simulink model "BatteryExampleUKF"  (R2017b)
settings: Solver=VariableStepAuto  StartTime=0.0  StopTime=100000  RelTol=1e-3
values from neighbouring files (symbols this model uses):
  C1_LUT = [1913.6 4625.7 23306 10736 18036 12251 9022.9 12447 18872 40764 18721 33630 ... (21 elements, 7x3)]    [BatteryParameters.mat]    (also in RW9_BatteryParameters.mat = [10000 10000 10000 10000 10000 10000 10000 9385.18668996 101)
  Capacity_LUT = [28.0081 27.625 27.6392]    [BatteryParameters.mat]    (also in RW9_BatteryParameters.mat = [2.6 2.55 2.5])
  cell_Cp_heat = 810.5328    [BatteryParameters.mat]    (also in RW9_BatteryParameters.mat = 35.3674127278)
  cell_mass = 1    [BatteryParameters.mat]    (also in RW9_BatteryParameters.mat = 0.0465)
  Em_LUT = [3.4966 3.5519 3.6183 3.7066 3.9131 4.0748 4.1923 3.5057 3.566 3.6337 3.7127 3.9259 ... (21 elements, 7x3)]    [BatteryParameters.mat]    (also in RW9_BatteryParameters.mat = [4 4 4 4 4 4 4 3.59172393305 3.73237152634 3.77937764301 3.8)
  InitCapacity = 30    [BatteryParameters.mat]    (also in RW9_BatteryParameters.mat = 2.6)
  LowerSOC = 0.3    [BatteryParameters.mat]    (also in RW9_BatteryParameters.mat)
  Qe_init = 15.6845    [BatteryParameters.mat]    (also in RW9_BatteryParameters.mat)
  R0_LUT = [0.0117 0.011 0.0114 0.0107 0.0107 0.0113 0.0116 0.0085 0.0085 0.0087 0.0082 0.0083 ... (21 elements, 7x3)]    [BatteryParameters.mat]    (also in RW9_BatteryParameters.mat = [0.1 0.1 0.1 0.1 0.1 0.1 0.1 0.129745781607 0.102359241178 0)
  R1_LUT = [0.0109 0.0069 0.0047 0.0034 0.0033 0.0033 0.0028 0.0029 0.0024 0.0026 0.0016 0.0023 ... (21 elements, 7x3)]    [BatteryParameters.mat]    (also in RW9_BatteryParameters.mat = [0.07 0.07 0.07 0.07 0.07 0.07 0.07 0.0768617046799 0.065453)
  SOC_LUT = [0 0.1 0.25 0.5 0.75 0.9 1]    [BatteryParameters.mat]    (also in RW9_BatteryParameters.mat)
  T_init = 293.15    [BatteryParameters.mat]    (also in RW9_BatteryParameters.mat)
  Temperature_LUT = [278.15 293.15 313.15]    [BatteryParameters.mat]    (also in RW9_BatteryParameters.mat)
  Ts = 1    [BatteryParameters.mat]    (also in RW9_BatteryParameters.mat)
  UpperSOC = 0.9    [BatteryParameters.mat]    (also in RW9_BatteryParameters.mat)
undefined symbols (not defined in the file or in its folder): DiscIntNeverNeededParam, Discrete, sigbuilder_block, Time
libraries: fl_lib x13, nesl_utility x8, simulink x5, ctrlSharedLib x1, sharedTrackingLibrary x1
settings Model: Creator=The MathWorks, Inc.  LastModifiedBy=imrenagi
settings CodeAppCC: StateflowObjectComments=on
settings SimscapeCC: SimscapeNormalizeSystem=off

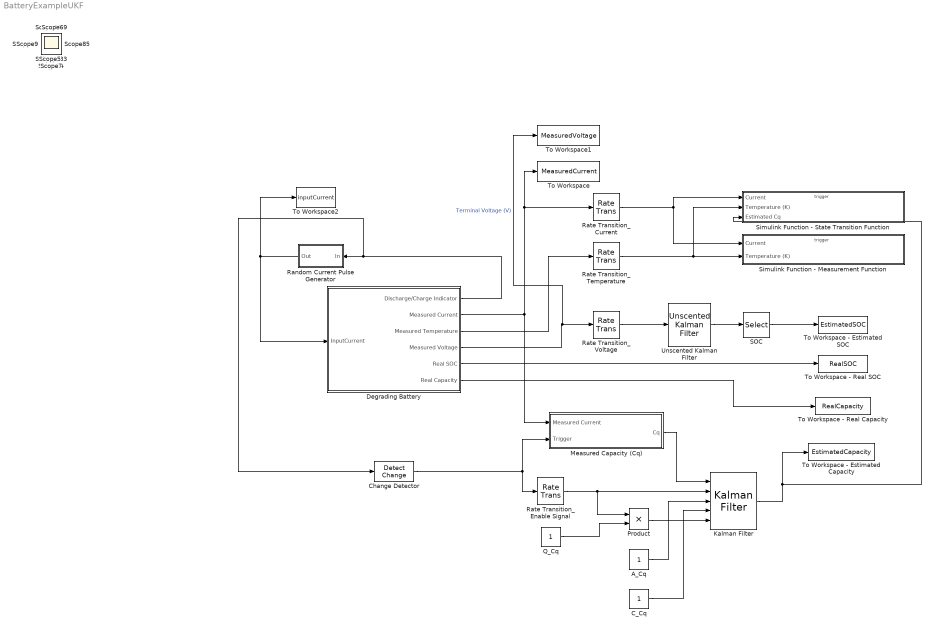
== system BatteryExampleUKF ==
  A_Cq : Constant
  C_Cq : Constant
  Change Detector : simulink/Logic and Bit Operations/Detect Change  vinit=-1  OutDataTypeStr=boolean
  Degrading Battery : Subsystem
  Kalman Filter : ctrlSharedLib/Kalman Filter  TimeDomain=Discrete-Time  UseCurrentEstimator=on  ModelSource=Input port  ModelSourceVariable=ss(0.95,1,1,0,1)  A=1  B=1  C=1  D=0  NumberOfStates=1  NumberOfInputs=1  NumberOfOutputs=1  InitialEstimateSource=Dialog  X0=2.6  P0=0.05  UseK=off  UseGH=off  NumberOfProcessNoiseInputs=1  G=1  TimeInvariantG=on  H=0  TimeInvariantH=on  Q=1  TimeInvariantQ=off  R=0.001  TimeInvariantR=on  N=0  TimeInvariantN=on  AddInputPort=off  AddEnablePort=on  OutputEstimatedY=off  OutputP=off  Ts=Ts
      settings: SourceProductBaseCode=CT
  Measured Capacity (Cq) : Subsystem
  Product : Product
  Q_Cq : Constant
  Random Current Pulse Generator : Subsystem
  Rate Transition_Current : RateTransition  OutPortSampleTime=Ts
  Rate Transition_Enable Signal : RateTransition  OutPortSampleTime=Ts
  Rate Transition_Temperature : RateTransition  InitialCondition=300  OutPortSampleTime=Ts
  Rate Transition_Voltage : RateTransition  InitialCondition=4  OutPortSampleTime=Ts
  SOC : Selector  InputPortWidth=2  IndexOptions=Index vector (dialog)  Indices=1  OutputSizes=1
  Simulink Function - Measurement Function : Subsystem  TreatAsAtomicUnit=on
  Simulink Function - State Transition Function : Subsystem  TreatAsAtomicUnit=on
  To Workspace : ToWorkspace  VariableName=MeasuredCurrent  SaveFormat=Timeseries  SampleTime=-1
  To Workspace - Estimated Capacity : ToWorkspace  VariableName=EstimatedCapacity  SaveFormat=Timeseries  SampleTime=-1
  To Workspace - Estimated SOC : ToWorkspace  VariableName=EstimatedSOC  SaveFormat=Timeseries  SampleTime=-1
  To Workspace - Real Capacity : ToWorkspace  VariableName=RealCapacity  SaveFormat=Timeseries  SampleTime=-1
  To Workspace - Real SOC : ToWorkspace  VariableName=RealSOC  SaveFormat=Timeseries  SampleTime=-1
  To Workspace1 : ToWorkspace  VariableName=MeasuredVoltage  SaveFormat=Timeseries  SampleTime=-1
  To Workspace2 : ToWorkspace  VariableName=inputCurrent  SaveFormat=Timeseries  SampleTime=-1
  Unscented Kalman Filter : sharedTrackingLibrary/Unscented Kalman Filter  StateTransitionFcn=batteryStateFcn  HasAdditiveProcessNoise=Additive  ProcessNoise=diag([2e-8, 3e-7])  HasTimeVaryingProcessNoise=off  HasStateTransitionFcnExtraArgument=0  InitialState=[1; 0]  InitialStateCovariance=diag([0.01, 1])  Alpha=1  Beta=2  Kappa=0  MeasurementFcn1=batteryMeasurementFcn  HasMeasurementEnablePort1=off  HasAdditiveMeasurementNoise1=Additive  MeasurementNoise1=1e-3  HasTimeVaryingMeasurementNoise1=off  HasMeasurementFcnExtraArgument1=0  MeasurementFcn2=myMeasurementFcn  HasMeasurementEnablePort2=off  HasAdditiveMeasurementNoise2=Additive  MeasurementNoise2=1  HasTimeVaryingMeasurementNoise2=off  HasMeasurementFcnExtraArgument2=0  MeasurementFcn3=myMeasurementFcn  HasMeasurementEnablePort3=off  HasAdditiveMeasurementNoise3=Additive  MeasurementNoise3=1  HasTimeVaryingMeasurementNoise3=off  HasMeasurementFcnExtraArgument3=0  MeasurementFcn4=myMeasurementFcn  HasMeasurementEnablePort4=off  HasAdditiveMeasurementNoise4=Additive  MeasurementNoise4=1  HasTimeVaryingMeasurementNoise4=off  HasMeasurementFcnExtraArgument4=0  MeasurementFcn5=myMeasurementFcn  HasMeasurementEnablePort5=off  HasAdditiveMeasurementNoise5=Additive  MeasurementNoise5=1  HasTimeVaryingMeasurementNoise5=off  HasMeasurementFcnExtraArgument5=0  EnableMultirate=off  StateTransitionFcnSampleTime=-1  MeasurementFcn1SampleTime=-1  MeasurementFcn2SampleTime=-1  MeasurementFcn3SampleTime=-1  MeasurementFcn4SampleTime=-1  MeasurementFcn5SampleTime=-1  UseCurrentEstimator=on  OutputStateCovariance=off  DataType=double  SampleTime=Ts  NumberOfMeasurements=1
      settings: SourceProductName=Control System Toolbox  SourceProductBaseCode=CT
  Scope{,1..11,13,17..18,20,22..35} (30 alike) : Scope
  wires:
  Degrading Battery/2(Measured Current) -> Measured Capacity (Cq)/1(Measured Current), To Workspace/1, Rate Transition_Current/1
  Rate Transition_Current/1 -> Simulink Function - Measurement Function/1(Current), Simulink Function - State Transition Function/1(Current)
  Unscented Kalman Filter/1 -> SOC/1
  Rate Transition_Voltage/1 -> Unscented Kalman Filter/1
  Rate Transition_Temperature/1 -> Simulink Function - State Transition Function/2(Temperature (K)), Simulink Function - Measurement Function/2(Temperature (K))
  Degrading Battery/1(Discharge/Charge Indicator) -> Change Detector/1, Random Current Pulse Generator/1(In)
  Random Current Pulse Generator/1(Out) -> To Workspace2/1, Degrading Battery/1(InputCurrent)
  SOC/1 -> To Workspace - Estimated SOC/1
  Degrading Battery/5(Real SOC) -> To Workspace - Real SOC/1
  Measured Capacity (Cq)/1(Cq) -> Kalman Filter/1
  Change Detector/1 -> Measured Capacity (Cq)/2(Trigger), Rate Transition_Enable Signal/1
  Kalman Filter/1 -> To Workspace - Estimated Capacity/1, Simulink Function - State Transition Function/3(Estimated Cq)
  Rate Transition_Enable Signal/1 -> Product/1, Kalman Filter/2
  Degrading Battery/3(Measured Temperature) -> Rate Transition_Temperature/1
  Degrading Battery/4(Measured Voltage) -> To Workspace1/1, Rate Transition_Voltage/1  "Terminal Voltage (V)"
  Product/1 -> Kalman Filter/5
  Q_Cq/1 -> Product/2
  A_Cq/1 -> Kalman Filter/3
  C_Cq/1 -> Kalman Filter/4
  Degrading Battery/6(Real Capacity) -> To Workspace - Real Capacity/1

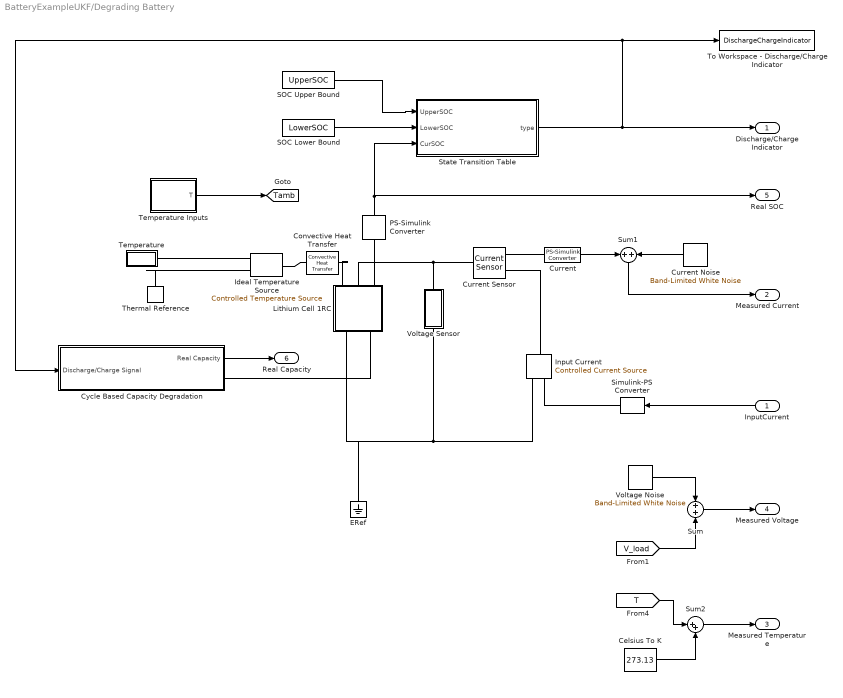
== system BatteryExampleUKF/Degrading Battery ==
  InputCurrent : Inport
  Celsius To K : Constant  Value=273.13
  Convective Heat Transfer : fl_lib/Thermal/Thermal Elements/Convective Heat Transfer  area=cell_area m^2  heat_tr_coeff=h_conv W/(m^2 * K)  T_specify=off  T_priority=High  T=0 K  T_nominal_specify=off  T_nominal_unit=K  T_nominal_value=1  Q_specify=off  Q_priority=High  Q=0 J/s  Q_nominal_specify=off  Q_nominal_unit=J/s  Q_nominal_value=1
  Current : nesl_utility/PS-Simulink Converter  PhysicalDomain=network_engine_domain  SubClassName=ps_output  LeftPortType=input  RightPortType=output  PseudoPeriodic=off  Frequencies=[]  Unit=1  AffineConversion=off
  Current Noise : simulink/Sources/Band-Limited White Noise  Cov=2.5e-2  Ts=Ts  seed=[1234]
  Current Sensor : fl_lib/Electrical/Electrical Sensors/Current Sensor
  Cycle Based Capacity Degradation : Subsystem
  ERef : fl_lib/Electrical/Electrical Elements/Electrical Reference
  Ideal Temperature Source : fl_lib/Thermal/Thermal Sources/Controlled Temperature Source
      settings: SourceProductName=Simscape
  Input Current : fl_lib/Electrical/Electrical Sources/Controlled Current Source
  Lithium Cell 1RC : Subsystem  Tag=PublishSubsystemCustomStyle  mask(Lithium cell (one RC-branch equivalent circuit)){Qe_init=Qe_init, T_init=T_init, Capacity_LUT=Capacity_LUT, Em_LUT=Em_LUT, R0_LUT=R0_LUT, R1_LUT=R1_LUT, C1_LUT=C1_LUT, cell_mass=cell_mass, cell_Cp_heat=cell_Cp_heat, SOC_LUT=SOC_LUT, Temperature_LUT=Temperature_LUT}
      mask prompts: Qe_init "Initial charge deficit (A*hr)"; T_init "Initial cell temperature (K)"; Capacity_LUT "Capacity (A*hr, 1xN table)"; Em_LUT "Em open-circuit voltage (volts, MxN table)"; R0_LUT "R0 terminal resistance (ohms, MxN table)"; R1_LUT "R1 resistance (ohms, MxN table)"; C1_LUT "C1 capacitance (farads, MxN table)"; cell_mass "Cell mass (kg)"; cell_Cp_heat "Cell specific heat (J/kg/K)"; SOC_LUT "SOC table breakpoints (Mx1 array)"; Temperature_LUT "Temperature table breakpoints (K, 1xN array)"
      mask DialogControl ParameterTabVar0 Prompt: Initial Conditions
      mask DialogControl ParameterTabVar01 Prompt: Electrical
      mask DialogControl ParameterTabVar012 Prompt: Thermal
      mask DialogControl ParameterTabVar0123 Prompt: Table Breakpoints
      mask Display:
      | % Battery icon
      | plot([0 0],[-1.5 -0.4])
      | plot([0 0 0.8 0.8],[0.2 0.9 0.9 1.5])
      | patch([-1 1 1 -1]*0.4,[1 1 -1 -1]*0.15-0.5,[0;0;0]);
      | patch([-1 1 1 -1]*0.9,[1 1 -1 -1]*0.15+0.1,[0;0;0]);
      | 
      | % Thermal port
      | plot([-1.2,-1.2],[0.5,0.9])
      | plot([-0.4,-0.4],[0.5,0.9])
      | plot([-0.8,-0.8],[0.9,1.5])
      | plot(0.35*cos(0:2*pi/50:2*pi)-0.8,0.15*sin(0:2*pi/50:2*pi)+0.85)
      | plot(0.35*cos(pi:2*pi/50:2*pi)-0.8,0.15*sin(pi:2*pi/50:2*pi)+0.55)
      | 
      | % Plot points to set plot range
      | color('white');plot(1.5,1.5);plot(-1.5,-1.5)
      | 
      | color('red')
      | port_label('LConn',1,'H')
      | port_label('LConn',2,'+')
      | port_label('RConn',1,'-')
  PS-Simulink Converter : nesl_utility/PS-Simulink Converter  PhysicalDomain=network_engine_domain  SubClassName=ps_output  LeftPortType=input  RightPortType=output  PseudoPeriodic=off  Frequencies=[]  Unit=1  AffineConversion=off
  SOC Lower Bound : Constant  Value=LowerSOC
  SOC Upper Bound : Constant  Value=UpperSOC
  Simulink-PS Converter : nesl_utility/Simulink-PS Converter  PhysicalDomain=network_engine_domain  SubClassName=ps_input  LeftPortType=input  RightPortType=output  PseudoPeriodic=off  Frequencies=[]  NoiseDistribution=none  NoiseParameters=[]  Unit=A  AffineConversion=off  FilteringAndDerivatives=zero  SimscapeFilterOrder=1  InputFilterTimeConstant=.001  UdotUserProvided=1
  State Transition Table : State Transition Table  TreatAsAtomicUnit=on
  Sum : Sum
  Sum1 : Sum
  Sum2 : Sum  Inputs=|++
  Temperature : Subsystem
      mask Display: disp('Tamb')
  Temperature Inputs : Subsystem
  Thermal Reference : fl_lib/Thermal/Thermal Elements/Thermal Reference
  To Workspace - Discharge/Charge Indicator : ToWorkspace  VariableName=DischargeChargeIndicator  SaveFormat=Timeseries  SampleTime=-1
  Voltage Sensor : Subsystem
      mask Display: disp('V_load')
  Voltage Noise : simulink/Sources/Band-Limited White Noise  Cov=1.5e-3  Ts=Ts  seed=[1234]
  Discharge/Charge Indicator : Outport
  Measured Current : Outport  Port=2
  Measured Temperature : Outport  Port=3
  Measured Voltage : Outport  Port=4
  Real SOC : Outport  Port=5
  Real Capacity : Outport  Port=6
  tag scope: Tamb=global
  wires:
  SOC Lower Bound/1 -> State Transition Table/2(LowerSOC)
  SOC Upper Bound/1 -> State Transition Table/1(UpperSOC)
  PS-Simulink Converter/1 -> State Transition Table/3(CurSOC), Real SOC/1
  Temperature Inputs/1(T) -> [Tamb]
  State Transition Table/1(type) -> To Workspace - Discharge/Charge Indicator/1, Cycle Based Capacity Degradation/1(Discharge/Charge Signal), Discharge/Charge Indicator/1
  [V_load] -> Sum/2
  Sum/1 -> Measured Voltage/1
  InputCurrent/1 -> Simulink-PS Converter/1
  Sum1/1 -> Measured Current/1
  Current/1 -> Sum1/1
  Current Noise/1 -> Sum1/2
  Celsius To K/1 -> Sum2/2
  Sum2/1 -> Measured Temperature/1
  [T] -> Sum2/1
  Cycle Based Capacity Degradation/1(Real Capacity) -> Real Capacity/1
  Voltage Noise/1 -> Sum/1
  connections:
  Lithium Cell 1RC/LConn1 -- Convective Heat Transfer/RConn1
  Current Sensor/RConn2 -- Input Current/LConn1
  Voltage Sensor/RConn1 -- Input Current/RConn2 -- ERef/LConn1 -- Lithium Cell 1RC/RConn1
  Lithium Cell 1RC/LConn3 -- PS-Simulink Converter/LConn1
  Current Sensor/LConn1 -- Lithium Cell 1RC/LConn2 -- Voltage Sensor/LConn1
  Current/LConn1 -- Current Sensor/RConn1
  Ideal Temperature Source/RConn1 -- Temperature/LConn1
  Ideal Temperature Source/RConn2 -- Thermal Reference/LConn1
  Simulink-PS Converter/RConn1 -- Input Current/RConn1
  Cycle Based Capacity Degradation/RConn1 -- Lithium Cell 1RC/RConn2
  Ideal Temperature Source/LConn1 -- Convective Heat Transfer/LConn1

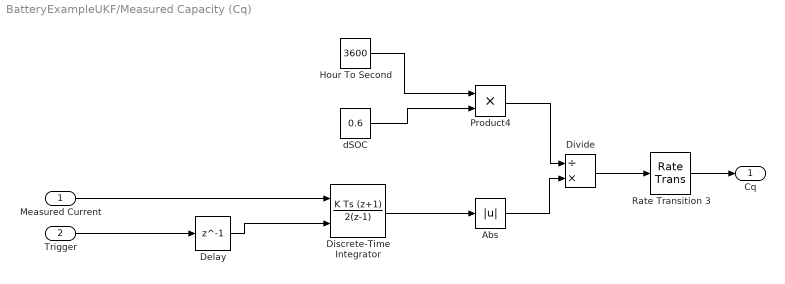
== system BatteryExampleUKF/Measured Capacity (Cq) ==
  Measured Current : Inport
  Trigger : Inport  Port=2
  Abs : Abs
  Delay : Delay  DelayLength=1  InitialCondition=0
  Discrete-Time Integrator : DiscreteIntegrator  IntegratorMethod=Integration: Trapezoidal  ExternalReset=rising  InitialConditionSetting=State (most efficient)  SampleTime=-1  ICPrevOutput=DiscIntNeverNeededParam  ICPrevScaledInput=DiscIntNeverNeededParam
  Divide : Product  Inputs=/*
  Hour To Second : Constant  Value=3600
  Product4 : Product
  Rate Transition 3 : RateTransition  InitialCondition=InitCapacity  OutPortSampleTime=Ts
  dSOC : Constant  Value=0.6
  Cq : Outport
  wires:
  Measured Current/1 -> Discrete-Time Integrator/1
  Abs/1 -> Divide/2
  Discrete-Time Integrator/1 -> Abs/1
  Product4/1 -> Divide/1
  Delay/1 -> Discrete-Time Integrator/2
  Hour To Second/1 -> Product4/1
  Trigger/1 -> Delay/1
  dSOC/1 -> Product4/2
  Rate Transition 3/1 -> Cq/1
  Divide/1 -> Rate Transition 3/1

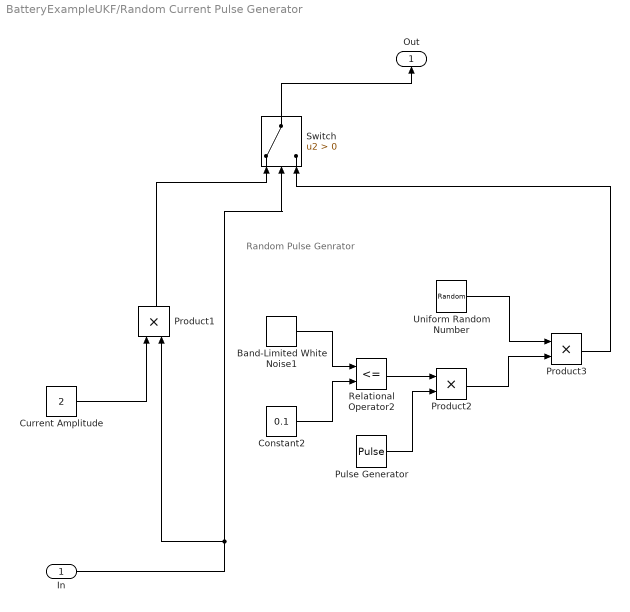
== system BatteryExampleUKF/Random Current Pulse Generator ==
  note: Random Pulse Genrator
  In : Inport
  Band-Limited White Noise1 : simulink/Sources/Band-Limited White Noise  Cov=0.1  Ts=50  seed=[23341]
  Constant2 : Constant  Value=0.1
  Current Amplitude : Constant  Value=2
  Product1 : Product
  Product2 : Product
  Product3 : Product
  Pulse Generator : DiscretePulseGenerator  PulseType=Time based  Amplitude=-1  Period=1000  PulseWidth=90
  Relational Operator2 : RelationalOperator  Operator=<=  OutDataTypeStr=boolean  RndMeth=Simplest
  Switch : Switch  Criteria=u2 > Threshold
  Uniform Random Number : UniformRandomNumber  Minimum=0.7  Maximum=1.5  SampleTime=100
  Out : Outport
  wires:
  In/1 -> Product1/2, Switch/2
  Constant2/1 -> Relational Operator2/2
  Band-Limited White Noise1/1 -> Relational Operator2/1
  Pulse Generator/1 -> Product2/2
  Relational Operator2/1 -> Product2/1
  Uniform Random Number/1 -> Product3/1
  Product2/1 -> Product3/2
  Product1/1 -> Switch/1
  Current Amplitude/1 -> Product1/1
  Product3/1 -> Switch/3
  Switch/1 -> Out/1

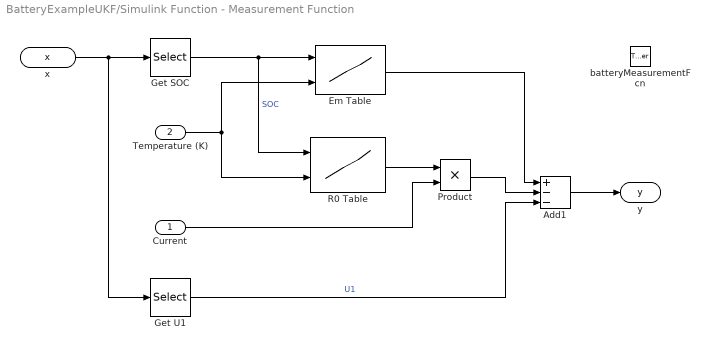
== system BatteryExampleUKF/Simulink Function - Measurement Function ==
  Current : Inport
  Temperature (K) : Inport  Port=2
  batteryMeasurementFcn : TriggerPort  TriggerType=function-call  IsSimulinkFunction=on  FunctionName=batteryMeasurementFcn  VariantControl=Variant
  Add1 : Sum  Inputs=+--
  Em Table : Lookup_n-D  BreakpointsForDimension1=SOC_LUT  BreakpointsForDimension2=Temperature_LUT  Table=Em_LUT  InternalRulePriority=Speed  RndMeth=Simplest  InputSameDT=on
  Get SOC : Selector  InputPortWidth=2  IndexOptions=Index vector (dialog)  Indices=[1]  OutputSizes=1
  Get U1 : Selector  InputPortWidth=2  IndexOptions=Index vector (dialog)  Indices=2  OutputSizes=1
  Product : Product
  R0 Table : Lookup_n-D  BreakpointsForDimension1=SOC_LUT  BreakpointsForDimension2=Temperature_LUT  Table=R0_LUT  InternalRulePriority=Speed  RndMeth=Simplest  InputSameDT=on
  x : ArgIn  DisableCoverage=on  PortDimensions=2  ArgumentName=x
  y : ArgOut  DisableCoverage=on  ArgumentName=y
  wires:
  x/1 -> Get U1/1, Get SOC/1
  Get SOC/1 -> R0 Table/1, Em Table/1  "SOC"
  Em Table/1 -> Add1/1
  Add1/1 -> y/1
  Temperature (K)/1 -> R0 Table/2, Em Table/2
  R0 Table/1 -> Product/1
  Current/1 -> Product/2
  Product/1 -> Add1/2
  Get U1/1 -> Add1/3  "U1"

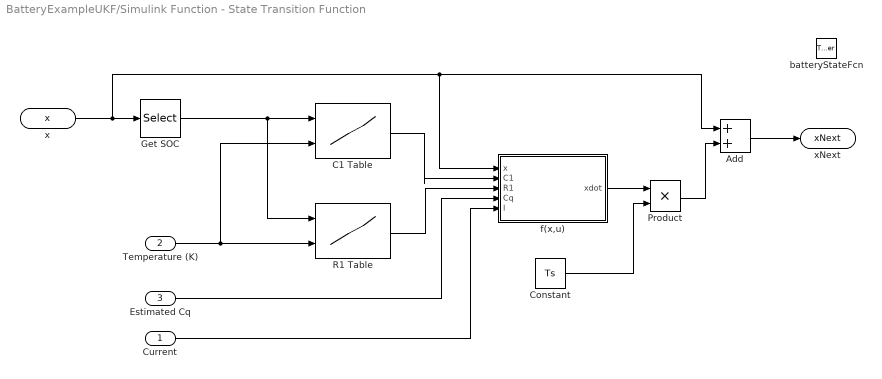
== system BatteryExampleUKF/Simulink Function - State Transition Function ==
  Current : Inport
  Temperature (K) : Inport  Port=2
  Estimated Cq : Inport  Port=3
  batteryStateFcn : TriggerPort  TriggerType=function-call  IsSimulinkFunction=on  FunctionName=batteryStateFcn  VariantControl=Variant
  Add : Sum
  C1 Table : Lookup_n-D  BreakpointsForDimension1=SOC_LUT  BreakpointsForDimension2=Temperature_LUT  Table=C1_LUT  InternalRulePriority=Speed  RndMeth=Simplest  InputSameDT=on
  Constant : Constant  Value=Ts
  Get SOC : Selector  InputPortWidth=2  IndexOptions=Index vector (dialog)  Indices=1  OutputSizes=1
  Product : Product
  R1 Table : Lookup_n-D  BreakpointsForDimension1=SOC_LUT  BreakpointsForDimension2=Temperature_LUT  Table=R1_LUT  InternalRulePriority=Speed  RndMeth=Simplest  InputSameDT=on
  f(x,u) : MATLAB Function  TreatAsAtomicUnit=on
  x : ArgIn  DisableCoverage=on  PortDimensions=2  ArgumentName=x
  xNext : ArgOut  DisableCoverage=on  PortDimensions=2  ArgumentName=xNext
  wires:
  x/1 -> f(x,u)/1(x), Add/1, Get SOC/1
  Add/1 -> xNext/1
  Temperature (K)/1 -> C1 Table/2, R1 Table/2
  Get SOC/1 -> R1 Table/1, C1 Table/1
  C1 Table/1 -> f(x,u)/2(C1)
  R1 Table/1 -> f(x,u)/3(R1)
  Current/1 -> f(x,u)/5(I)
  Constant/1 -> Product/2
  f(x,u)/1(xdot) -> Product/1
  Product/1 -> Add/2
  Estimated Cq/1 -> f(x,u)/4(Cq)

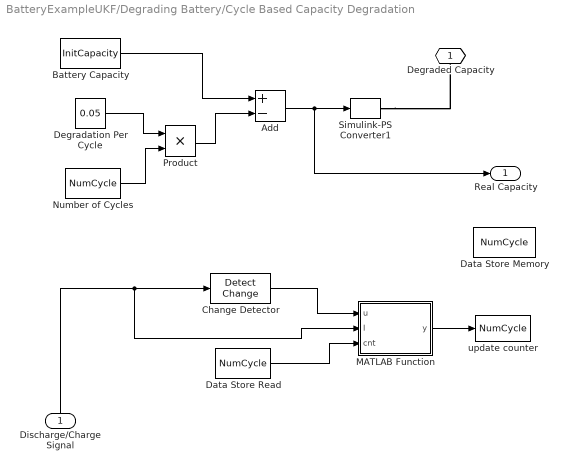
== system BatteryExampleUKF/Degrading Battery/Cycle Based Capacity Degradation ==
  Discharge/Charge Signal : Inport
  Add : Sum  Inputs=+-
  Battery Capacity : Constant  Value=InitCapacity
  Change Detector : simulink/Logic and Bit Operations/Detect Change  vinit=-1  OutDataTypeStr=boolean
  Data Store Memory : DataStoreMemory  DataStoreName=NumCycle  ShowAdditionalParam=off
  Data Store Read : DataStoreRead  DataStoreName=NumCycle
  Degradation Per Cycle : Constant  Value=0.05
  MATLAB Function : MATLAB Function  TreatAsAtomicUnit=on
  Number of Cycles : DataStoreRead  DataStoreName=NumCycle
  Product : Product
  Simulink-PS Converter1 : nesl_utility/Simulink-PS Converter  PhysicalDomain=network_engine_domain  SubClassName=ps_input  LeftPortType=input  RightPortType=output  PseudoPeriodic=off  Frequencies=[]  NoiseDistribution=none  NoiseParameters=[]  Unit=hr*A  AffineConversion=off  FilteringAndDerivatives=zero  SimscapeFilterOrder=1  InputFilterTimeConstant=.001  UdotUserProvided=1
  update counter : DataStoreWrite  DataStoreName=NumCycle
  Degraded Capacity : PMIOPort  Port=1  Side=Right
  Real Capacity : Outport
  wires:
  Add/1 -> Real Capacity/1, Simulink-PS Converter1/1
  Degradation Per Cycle/1 -> Product/1
  MATLAB Function/1(y) -> update counter/1
  Battery Capacity/1 -> Add/1
  Change Detector/1 -> MATLAB Function/1(u)
  Number of Cycles/1 -> Product/2
  Product/1 -> Add/2
  Data Store Read/1 -> MATLAB Function/3(cnt)
  Discharge/Charge Signal/1 -> Change Detector/1, MATLAB Function/2(I)
  connections:
  Simulink-PS Converter1/RConn1 -- Degraded Capacity/RConn1

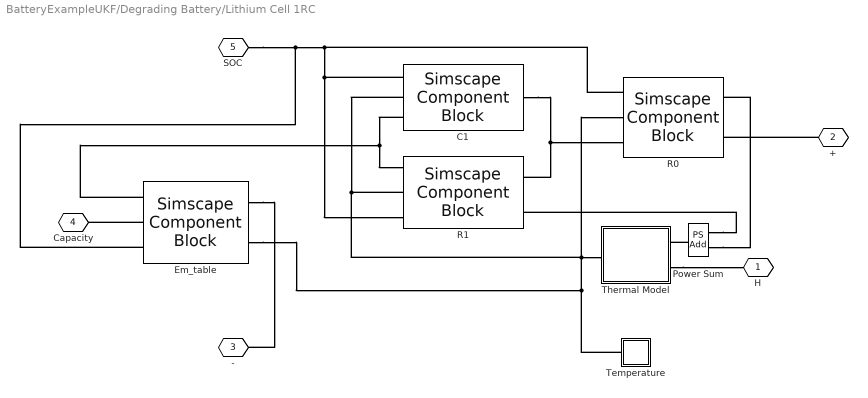
== system BatteryExampleUKF/Degrading Battery/Lithium Cell 1RC ==
  C1 : SimscapeComponentBlock  SourceFile=C_table  ComponentPath=C_table  ComponentVariants=C_table  ComponentVariantNames=C_table  ClassName=C_table  SchemaVersion=1  C_Table=C1_LUT F  SOC_Table=SOC_LUT  Temp_Table=Temperature_LUT K  v0=0 V
      settings: CopyFcn=simscape.engine.sli.internal.componentblockcallback(gcbh,'COPY')  PreCopyFcn=simscape.engine.sli.internal.componentblockcallback(gcbh,'PRECOPY')  PreDeleteFcn=simscape.engine.sli.internal.componentblockcallback(gcbh,'PREDELETE')
      mask Type: C_table
      mask Display:
      | disp('Simscape\n\n\n')
      | disp('\n\n\nC_table');
      | color('red');
      | port_label('LConn', 3,'SOC');
      | port_label('LConn', 2,'T');
      | port_label('RConn', 1,'-');
      | port_label('LConn', 1,'+');
  Em_table : SimscapeComponentBlock  SourceFile=Em_table  ComponentPath=Em_table  ComponentVariants=Em_table  ComponentVariantNames=Em_table  ClassName=Em_table  SchemaVersion=1  Em_Table=Em_LUT V  SOC_Table=SOC_LUT  Temp_Table=Temperature_LUT K  Qinit=Qinit hr*A
      settings: CopyFcn=simscape.engine.sli.internal.componentblockcallback(gcbh,'COPY')  PreCopyFcn=simscape.engine.sli.internal.componentblockcallback(gcbh,'PRECOPY')  PreDeleteFcn=simscape.engine.sli.internal.componentblockcallback(gcbh,'PREDELETE')
      mask Type: Em_table
      mask Display:
      | disp('Simscape\n\n\n')
      | disp('\n\n\nEm_table');
      | color('red');
      | port_label('LConn', 3,'SOC');
      | port_label('LConn', 2,'Capacity');
      | port_label('RConn', 2,'T');
      | port_label('RConn', 1,'-');
      | port_label('LConn', 1,'+');
  Power Sum : fl_lib/Physical Signals/Functions/PS Add
  R0 : SimscapeComponentBlock  SourceFile=R_table  ComponentPath=R_table  ComponentVariants=R_table  ComponentVariantNames=R_table  ClassName=R_table  SchemaVersion=1  R_Table=R0_LUT Ohm  SOC_Table=SOC_LUT  Temp_Table=Temperature_LUT K
      settings: CopyFcn=simscape.engine.sli.internal.componentblockcallback(gcbh,'COPY')  PreCopyFcn=simscape.engine.sli.internal.componentblockcallback(gcbh,'PRECOPY')  PreDeleteFcn=simscape.engine.sli.internal.componentblockcallback(gcbh,'PREDELETE')
      mask Type: R_table
      mask Display:
      | disp('Simscape\n\n\n')
      | disp('\n\n\nR_table');
      | color('red');
      | port_label('RConn', 2,'POW');
      | port_label('LConn', 3,'SOC');
      | port_label('LConn', 2,'T');
      | port_label('RConn', 1,'-');
      | port_label('LConn', 1,'+');
  R1 : SimscapeComponentBlock  SourceFile=R_table  ComponentPath=R_table  ComponentVariants=R_table  ComponentVariantNames=R_table  ClassName=R_table  SchemaVersion=1  R_Table=R1_LUT Ohm  SOC_Table=SOC_LUT  Temp_Table=Temperature_LUT K
      settings: CopyFcn=simscape.engine.sli.internal.componentblockcallback(gcbh,'COPY')  PreCopyFcn=simscape.engine.sli.internal.componentblockcallback(gcbh,'PRECOPY')  PreDeleteFcn=simscape.engine.sli.internal.componentblockcallback(gcbh,'PREDELETE')
      mask Type: R_table
      mask Display:
      | disp('Simscape\n\n\n')
      | disp('\n\n\nR_table');
      | color('red');
      | port_label('RConn', 2,'POW');
      | port_label('LConn', 3,'SOC');
      | port_label('LConn', 2,'T');
      | port_label('RConn', 1,'-');
      | port_label('LConn', 1,'+');
  Temperature : Subsystem
  Thermal Model : Subsystem
  H : PMIOPort  Tag=PMCPort  Port=1  Side=Left
  + : PMIOPort  Tag=PMCPort  Port=2  Side=Left
  - : PMIOPort  Tag=PMCPort  Port=3  Side=Right
  Capacity : PMIOPort  Tag=PMCPort  Port=4  Side=Right
  SOC : PMIOPort  Tag=PMCPort  Port=5  Side=Left
  connections:
  R0/LConn3 -- Em_table/LConn3 -- SOC/RConn1 -- R1/LConn3 -- C1/LConn3
  Thermal Model/LConn2 -- H/RConn1
  Em_table/RConn1 -- -/RConn1
  +/RConn1 -- R0/RConn1
  C1/LConn1 -- R1/LConn1 -- Em_table/LConn1
  Power Sum/LConn2 -- R1/RConn2
  R0/LConn2 -- Em_table/RConn2 -- Temperature/LConn1 -- Thermal Model/RConn1 -- R1/LConn2 -- C1/LConn2
  Power Sum/RConn1 -- Thermal Model/LConn1
  C1/RConn1 -- R1/RConn1 -- R0/LConn1
  Power Sum/LConn1 -- R0/RConn2
  Em_table/LConn2 -- Capacity/RConn1

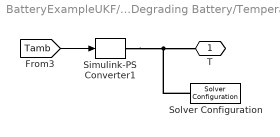
== system BatteryExampleUKF/Degrading Battery/Temperature ==
  Simulink-PS Converter1 : nesl_utility/Simulink-PS Converter  PhysicalDomain=network_engine_domain  SubClassName=ps_input  LeftPortType=input  RightPortType=output  PseudoPeriodic=off  Frequencies=[]  NoiseDistribution=none  NoiseParameters=[]  Unit=degC  AffineConversion=on  FilteringAndDerivatives=zero  SimscapeFilterOrder=1  InputFilterTimeConstant=.001  UdotUserProvided=1
  Solver Configuration : nesl_utility/Solver Configuration  PhysicalDomain=network_engine_domain  SubClassName=solver  LeftPortType=input  RightPortType=generic  Accelerate=off  Tones=[]  Harmonics=[]  SimulateNoise=off  Profile=off  UseLocalSampling=off  EnableSwitchedLinearOptims=on  FrequencyDomain=off  UseCCode=off  RelTol=0.001  AbsTol=1e-06  MinStep=1e-09  ToWorkspace=off  RevertToSquareIcSolve=off  NumHomotopyIterations=100  PhasorMode=off  PhasorModeNumHarmonics=1  DoDC=off  ResidualTolerance=1e-9  UseLocalSolver=off  LocalSolverChoice=NE_BACKWARD_EULER_ADVANCER  LocalSolverSampleTime=1  DoFixedCost=off  MaxNonlinIter=3  MaxModeIter=2  LinearAlgebra=Sparse  DelaysMemoryBudget=1024  AutomaticFiltering=on  FilteringTimeConstant=0.001
  T : PMIOPort  Port=1  Side=Left
  wires:
  [Tamb] -> Simulink-PS Converter1/1
  connections:
  Simulink-PS Converter1/RConn1 -- Solver Configuration/RConn1 -- T/RConn1

== system BatteryExampleUKF/Degrading Battery/Temperature Inputs ==
  Signal Builder : Subsystem  Tag=STV Subsys  LoadFcn=sigbuilder_block('load');  StartFcn=sigbuilder_block('start');  StopFcn=sigbuilder_block('stop');  ClipboardFcn=sigbuilder_block('clipboard');  mask(Sigbuilder block){tuvar=[0:10]}
      mask help: Simulink:masks:SigbuilderBlock_MD
      mask init:
      | if ~strcmp(get_param(bdroot(gcbh),'SimulationStatus'),'stopped') tuvar = sigbuilder_block('maskInit'); end
      settings: CopyFcn=sigbuilder_block('copy');  DeleteFcn=sigbuilder_block('delete');  ModelCloseFcn=sigbuilder_block('modelClose');  PreSaveFcn=sigbuilder_block('preSave');  PauseFcn=sigbuilder_block('pause');  ContinueFcn=sigbuilder_block('continue');  NameChangeFcn=sigbuilder_block('namechange');  OpenFcn=sigbuilder_block('open',[45.75 269.25 978 385.5 ]);  CloseFcn=sigbuilder_block('close');
      mask Display: plot(0, 0, 100, 100,[2, 2, 32, 32, 2], [68, 8, 8, 68, 68],[32, 2], [38, 38], [32, 19, 2],[53, 60, 44], [32, 17, 17, 2],[16, 16, 31, 31]);txt = getActiveGroup(gcbh);text(2, 100, txt,'verticalAlignment', 'top');
  T : Outport
  wires:
  Signal Builder/1(Ambient Temp) -> T/1

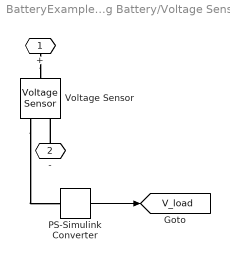
== system BatteryExampleUKF/Degrading Battery/Voltage Sensor ==
  PS-Simulink Converter : nesl_utility/PS-Simulink Converter  PhysicalDomain=network_engine_domain  SubClassName=ps_output  LeftPortType=input  RightPortType=output  PseudoPeriodic=off  Frequencies=[]  Unit=V  AffineConversion=off
  Voltage Sensor : fl_lib/Electrical/Electrical Sensors/Voltage Sensor
  + : PMIOPort  Port=1  Side=Left
  - : PMIOPort  Port=2  Side=Right
  tag scope: V_load=global
  wires:
  PS-Simulink Converter/1 -> [V_load]
  connections:
  Voltage Sensor/RConn1 -- PS-Simulink Converter/LConn1
  +/RConn1 -- Voltage Sensor/LConn1
  -/RConn1 -- Voltage Sensor/RConn2

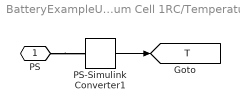
== system BatteryExampleUKF/Degrading Battery/Lithium Cell 1RC/Temperature ==
  PS-Simulink Converter1 : nesl_utility/PS-Simulink Converter  PhysicalDomain=network_engine_domain  SubClassName=ps_output  LeftPortType=input  RightPortType=output  PseudoPeriodic=off  Frequencies=[]  Unit=degC  AffineConversion=on
  PS : PMIOPort  Port=1  Side=Left
  tag scope: T=global
  wires:
  PS-Simulink Converter1/1 -> [T]
  connections:
  PS/RConn1 -- PS-Simulink Converter1/LConn1

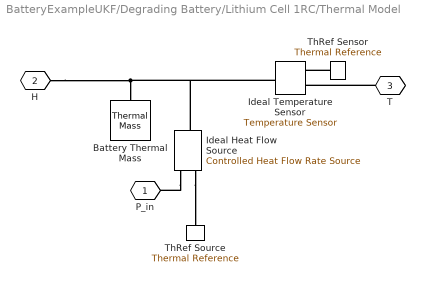
== system BatteryExampleUKF/Degrading Battery/Lithium Cell 1RC/Thermal Model ==
  Battery Thermal Mass : fl_lib/Thermal/Thermal Elements/Thermal Mass  mass=cell_mass kg  sp_heat=cell_Cp_heat J/kg/K  T_specify=on  T_priority=High  T=T_init K  T_nominal_specify=off  T_nominal_unit=K  T_nominal_value=1  Q_specify=off  Q_priority=High  Q=0 J/s  Q_nominal_specify=off  Q_nominal_unit=J/s  Q_nominal_value=1
  Ideal Heat Flow Source : fl_lib/Thermal/Thermal Sources/Controlled Heat Flow Rate Source
      settings: SourceProductName=Simscape
  Ideal Temperature Sensor : fl_lib/Thermal/Thermal Sensors/Temperature Sensor
  ThRef Sensor : fl_lib/Thermal/Thermal Elements/Thermal Reference
  ThRef Source : fl_lib/Thermal/Thermal Elements/Thermal Reference
  P_in : PMIOPort  Tag=PMCPort  Port=1  Side=Left
  H : PMIOPort  Tag=PMCPort  Port=2  Side=Left
  T : PMIOPort  Tag=PMCPort  Port=3  Side=Right
  connections:
  ThRef Sensor/LConn1 -- Ideal Temperature Sensor/RConn1
  T/RConn1 -- Ideal Temperature Sensor/RConn2
  Ideal Heat Flow Source/RConn2 -- ThRef Source/LConn1
  Ideal Temperature Sensor/LConn1 -- Ideal Heat Flow Source/LConn1 -- H/RConn1 -- Battery Thermal Mass/LConn1
  Ideal Heat Flow Source/RConn1 -- P_in/RConn1

== system BatteryExampleUKF/Degrading Battery/Temperature Inputs/Signal Builder ==
  Demux : Demux  Tag=STV Demux  Outputs=1
  FromWs : FromWorkspace  Tag=STV FromWs  VariableName=tuvar  SampleTime=0
      SigBuilderData=|
      | common.afterFinalStr = 'Extrapolate'
      | common.sampleTime = 0
      | dataSet(1).timeRange = [0 40000]
      | dataSet(1).name = 'Pulse'
      | dataSet(2).timeRange = [0 40000]
      | dataSet(2).name = 'Constant'
      | sbobj.Name = 'Signal Builder'
      | sbobj.Groups(1).Name = 'Pulse'
      | sbobj.Groups(1).Signals.Name = 'Ambient Temp'
      | sbobj.Groups(1).Signals.XData = [0 300 2100 3600 3960 7200 7560 10800 11160 14400 14760 18000 18360 21600 21960 25200 25560 28800 29160 32400 32760 36000 36360 40000]
      | sbobj.Groups(1).Signals.YData = [20 20 20 20 20 20 20 20 20 20 20 20 20 20 20 20 20 20 20 20 20 20 20 20]
      | sbobj.Groups(1).TimeRange = [0 40000]
      | sbobj.Groups(2).Name = 'Constant'
      | sbobj.Groups(2).Signals.Name = 'Ambient Temp'
      | sbobj.Groups(2).Signals.XData = [0 360 9100 11800 28200 33800 40000]
      | sbobj.Groups(2).Signals.YData = [20 20.09 22.275 22.95 27.05 28.45 30]
      | sbobj.Groups(2).TimeRange = [0 40000]
  Ambient Temp : Outport  Tag=STV Outport
  wires:
  FromWs/1 -> Demux/1
  Demux/1 -> Ambient Temp/1

== matlab function BatteryExampleUKF/Simulink Function - State Transition Function/f(x,u) ==
  data: x input; C1 input; R1 input; Cq input; I input; xdot output
function xdot = fx(x,C1,R1,Cq,I)
xdot = zeros(size(x));
U1 = x(2);
xdot(1) = -I/(3600*Cq);
xdot(2) = -1/(R1*C1)*U1 + I/C1;

== stateflow chart BatteryExampleUKF/Degrading Battery/State Transition Table ==
  settings: stateMachineType=MOORE_MACHINE
  state Discharge
    type = -1.0;
  state Charge
    type = 1.0;
  (default) -> Discharge
  Discharge -> (junction 166) [order 1] : [CurSOC>LowerSOC]
  (junction 166) -> Discharge
  Discharge -> Charge [order 2]
  Charge -> Discharge [order 2]
  Charge -> (junction 170) [order 1] : [CurSOC<UpperSOC]
  (junction 170) -> Charge
  data: type output =-1; UpperSOC input; LowerSOC input; CurSOC input

== matlab function BatteryExampleUKF/Degrading Battery/Cycle Based Capacity Degradation/MATLAB Function ==
  data: u input; I input; y output; cnt input
function y = fcn(u,I,cnt)

if(u>=1 && I<0)
    cnt = cnt+1;
end
y = cnt;
